simulink model "AM_DSB_TC_PLL"  (R2014b)
settings: Solver=VariableStepDiscrete  StartTime=0.0  StopTime=10  RelTol=1e-3
PreLoadFcn:
  | %%%%%%%%%%%%%%%%%%%%%%%%%%%%%%%%%%%%%%%%%%%%%%%%%%%%%%%%%%%%%%%%%%%%%%%%%%%
  | % check to see if Simulink library folder is missing from the MATLAB path %
  | %%%%%%%%%%%%%%%%%%%%%%%%%%%%%%%%%%%%%%%%%%%%%%%%%%%%%%%%%%%%%%%%%%%%%%%%%%%
  | if isempty(strfind(path, 'rtlsdr_book_library'))
  | 
  |     % create error window
  |     fig_error = figure(...
  |         'Name', 'Error: RTL-SDR Book Library',...
  |         'Toolbar','none',...
  |         'MenuBar','none',...
  |         'NumberTitle','off',...
  |         'Resize','off',...
  |         'WindowStyle','modal');
  |     fig_error.Position(3) = 600;
  |     fig_error.Position(4) = 150;
  |     fig_axes = axes(...
  |         'Parent',fig_error,...
  |         'Position',[0,0,1,1],...
  |         'visible','off');
  |     % error message
  |     t_title = text(.05,.8,...
  |         'MISSING DIRECTORIES',...
  |         'FontSize',11.5);
  |     t_body = text(.075,.6,...
  |         [{'Simulink cannot find the  \it{<root>}\rm / \it{rtlsdr\_book\_library}\rm  folder in the \it{MATLAB Path}\rm.'},...
  |         {'Please set the MATLAB path following the instructions given in Exercise 2.4.'}],...
  |         'FontSize',10.5);
  |     % buttons
  |     btn_path = uicontrol(...
  |         'Parent',fig_error,...
  |         'String','Set Path Now',...
  |         'FontSize',10,...
  |         'Callback', 'pathtool; close(fig_error);',...
  |         'Position', [fig_error.Position(3)/2-210, 30, 200, 30]);
  |     btn_abort = uicontrol(...
  |         'Parent',fig_error,...
  |         'String','No thanks',...
  |         'FontSize',10,...
  |         'Callback', 'close(fig_error); abort=1;',...
  |         'Position', [fig_error.Position(3)/2+10, 30, 200, 30]);
  | 
  |     % pause to allow user to interact with error box
  |     uiwait(fig_error);
  | 
  |     % abort simulation
  |     try
  |         if abort==1
  |             set_param(gcs, 'SimulationCommand', 'stop');
  |         end
  |     end
  | 
  |     % if user has set path, allow diagram to be updated
  |     if ~exist('abort','var')
  |         % create error window
  |         fig_update = figure(...
  |             'Name', 'Update Diagram',...
  |             'Toolbar','none',...
  |             'MenuBar','none',...
  |             'NumberTitle','off',...
  |             'Resize','off');
  |         fig_update.Position(3) = 400;
  |         fig_update.Position(4) = 120;
  |         fig_axes = axes(...
  |             'Parent',fig_update,...
  |             'Position',[0,0,1,1],...
  |             'visible','off');
  |         % instruction message
  |         t_body = text(.075,.7,...
  |             'Once you have set the path, update the block diagram',...
  |             'FontSize',10.5);
  |         % button
  |         btn_update = uicontrol(...
  |             'Parent',fig_update,...
  |             'String','Update Block Diagram',...
  |             'FontSize',10,...
  |             'Callback', 'set_param(gcs,''SimulationCommand'',''update''); close(gcf)',...
  |             'Position', [fig_update.Position(3)/2-100, 30, 200, 30]);
  |     end
  | 
  |     % clear error components
  |     clear('fig_error','fig_update','fig_axes','t_title','t_body','btn_path','btn_abort','btn_update','abort');
  | 
  | end
  | %%%%%%%%%%%%%%%%%%%%%%%%%%%%%%%%%%%%%%%%%%%%%%%%%%%%%%%%%%%%%%%%%%%%%%%%%%%
  | 
  | 
  | fs = 48e3*10;
  | kHz = fs/1000;
  | 
  | fc = fs/5;
  | 
  | % ------- section for synch loop design --------
  | 
  | A = 1;          % assume amplitude of input to PD is 1
  | 
  | T = 1/fs;       % sample period
  | Kp = A/2;      % phase detector is a multiplier
  | Bn = 1000;     % noise bandwidth in Hz
  | Ko = 1;         % gain of NCO (normalised to fs)
  | 
  | d = 0.707;  % damping ratio
  | 
  | % calculate the loop filter coefficients
  | K1 = (4*d*Bn*T)/(Ko*Kp*(d+1/(4*d)));
  | K2 = (4*(Bn*T)^2)/(Ko*Kp*(d+1/4*d)^2);
StopFcn:
  | figure(1)
  | hold off;
  | plot(tx_freq.time,tx_freq.signals.values,'r');
  | hold on;
  | grid on;
  | plot(lo_freq.time,lo_freq.signals.values,'b');
  | xlabel('Time (seconds)');
  | ylabel('Synthesised Frequency (Hz)');
  | legend('Transmitted Carrier','Locally Generated Carrier','location','NorthEast');
  | set(1,'Name','Frequencies of Transmitted and Locally Generated Carriers','NumberTitle','off');
  | setStandardFigSize(1);
undefined symbols (not defined in the file): startfcn_time_scope
libraries: dspmlti4 x6, dspvision x2, commsynccomp2 x2, dsparch4 x1, rtlsdr_book_library x1
CloseFcn:
  | closefcn_model;
Description:
  | Software, Simulation Examples and Design Exercises Licence Agreement
  | 
  | This license agreement refers to the simulation examples, design exercises and files,
  | and associated software MATLAB and Simulink resources that accompany the book:
  | 
  |      Title: Software Defined Radio using MATLAB & Simulink and the RTL-SDR
  |      Published by Strathclyde Academic Media, 2015
  |      Authored by Robert W. Stewart, Kenneth W. Barlee, Dale S.W. Atkinson,
  |      and Louise H. Crockett
  | 
  | and made available as a download from, www.desktopSDR.com or variously acquired
  | by other means such as via USB storage, cloud storage, disk or any other electronic
  | or optical or magnetic storage mechanism. These files and associated software may
  | be used subject to the terms of agreement of the conditions below:
  | 
  |     Copyright © 2015 Robert W. Stewart, Kenneth W. Barlee, Dale S.W. Atkinson,
  |     and Louise H. Crockett
  |     All rights reserved.
  | 
  | Redistribution and use in source and binary forms, with or without modification, are
  | permitted provided that the following conditions are met:
  | 
  |    1.  Redistributions of source code must retain the above copyright notice, this list of
  |         conditions and the following disclaimer.
  | 
  |    2.  Redistributions in binary form must reproduce the above copyright notice, this
  |         list of conditions and the following disclaimer in the documentation and/or other
  |         materials provided with the distribution.
  | 
  |    3.  Neither the name of the copyright holder nor the names of its contributors may
  |         be used to endorse or promote products derived from this software without
  |         specific prior written permission.
  | 
  |    4.  In all cases, the software is, and all modifications and derivatives of the
  |         software shall be, licensed to you solely for use in conjunction with The
  |         MathWorks, Inc. products and service offerings.
  | 
  | THIS SOFTWARE IS PROVIDED BY THE COPYRIGHT HOLDERS AND CONTRIBUTORS
  | "AS IS" AND ANY EXPRESS OR IMPLIED WARRANTIES, INCLUDING, BUT NOT LIMITED
  | TO, THE IMPLIED WARRANTIES OF MERCHANTABILITY AND FITNESS FOR A
  | PARTICULAR PURPOSE ARE DISCLAIMED. IN NO EVENT SHALL THE COPYRIGHT
  | HOLDER OR CONTRIBUTORS BE LIABLE FOR ANY DIRECT, INDIRECT, INCIDENTAL,
  | SPECIAL, EXEMPLARY, OR CONSEQUENTIAL DAMAGES (INCLUDING, BUT NOT
  | LIMITED TO, PROCUREMENT OF SUBSTITUTE GOODS OR SERVICES; LOSS OF USE,
  | DATA, OR PROFITS; OR BUSINESS INTERRUPTION) HOWEVER CAUSED AND ON ANY
  | THEORY OF LIABILITY, WHETHER IN CONTRACT, STRICT LIABILITY, OR TORT
  | (INCLUDING NEGLIGENCE OR OTHERWISE) ARISING IN ANY WAY OUT OF THE USE
  | OF THIS SOFTWARE, EVEN IF ADVISED OF THE POSSIBILITY OF SUCH DAMAGE.
  | 
  | 
  | Audio Tracks used in Simulations Examples and Design Exercises
  | 
  | The music and vocal files used within the Examples files and software within the book
  | were variously written, arranged, performed, recorded and produced by Garrey Rice,
  | Adam Struth, Jamie Struth, Iain Thistlethwaite and also Marshall Craigmyle who
  | collectively, and individually where appropriate, assert and retain all of their copyright,
  | performance and artistic rights. Permission to use and reproduce this music is
  | granted for all purposes associated with MATLAB and Simulink software and the
  | simulation examples and design exercises files that accompany this book. Requests to
  | use the music for any other purpose should be directed to: info@desktopSDR.com.
  | For information on music track names, full credits, and links to the musicians please
  | refer to www.desktopSDR.com/more/audio.
settings Model: Creator=desktopSDR Team  LastModifiedBy=desktopSDR Team
settings DataIOCC: LimitDataPoints=off  SaveOutput=off  SignalLogging=off  SaveTime=off
settings OptimizationCC: InlineParams=on
settings DebuggingCC: ReadBeforeWriteMsg=DisableAll  WriteAfterWriteMsg=DisableAll  WriteAfterReadMsg=DisableAll  UnderspecifiedInitializationDetection=Classic  MergeDetectMultiDrivingBlocksExec=none  MultiTaskDSMMsg=none  ParameterPrecisionLossMsg=none
settings ModelReferenceCC: UpdateModelReferenceTargets=IfOutOfDate
settings SFSimCC: SFSimEcho=off

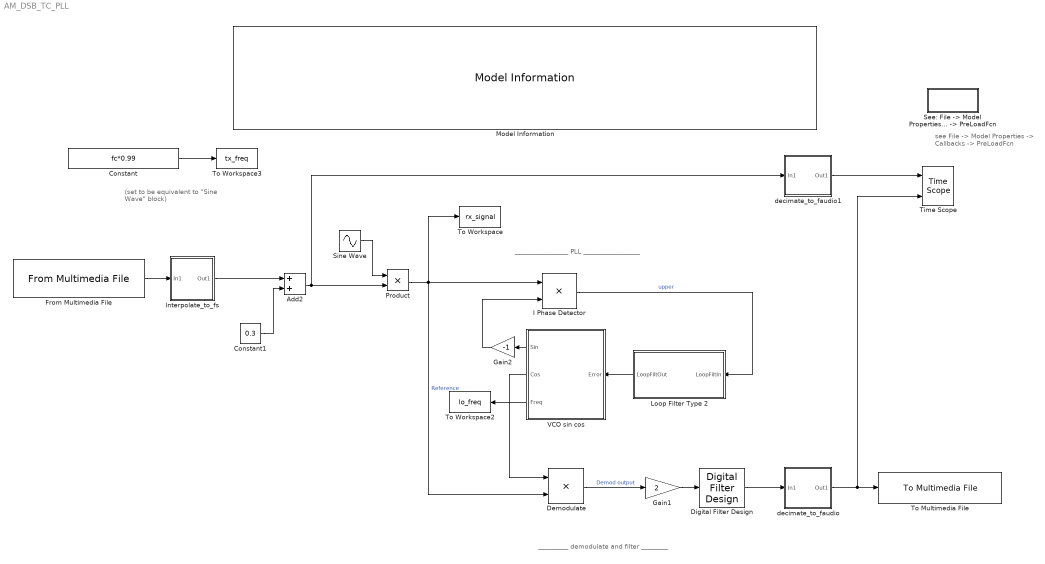
== system AM_DSB_TC_PLL ==
  note: (set to be equivalent to
      | "Sine Wave" block)
  note: ________________ PLL _________________
  note: see File -> Model Properties
      | -> Callbacks -> PreLoadFcn
  note: _________ demodulate and filter ________
  Add2 : Sum
  Constant : Constant  Value=fc*0.99  SampleTime=1/fs
  Constant1 : Constant  Value=0.3  SampleTime=1/fs
  Demodulate : Product
  Digital Filter Design : dsparch4/Digital Filter Design  mwdsp_browser_bugfix_var=off
  From Multimedia File : dspvision/From Multimedia File  inputFilename=..\..\audio_sources\music1_mono48kHz.wav  loop=on  numPlays=inf  outputStreams=Audio only  videoDataType=single  audioDataType=double  inheritSampleTime=on  userDefinedSampleTime=1/30  noAudioOutput=off  isIntensityVideo=off  fourcc=RGB  colorVideoFormat=Separate color signals  outputEOF=off  dataOrg=Column-major  audioFrameSize=600  computeAudioFrameSize=off  outSamplingMode=Frame based
  Gain1 : Gain  Gain=2
  Gain2 : Gain  Gain=-1
  I Phase Detector : Product
  Interpolate_to_fs : Subsystem
  Loop Filter Type 2 : Subsystem  mask(Loop Filter (Type 2)){K1=K1, K2=K2}
      mask prompts: K1 "K1 (proportional path)"; K2 "K2 (integral path)"
      mask help: This loop filter contains two paths: a proportional path with scaling coefficient K1, and an integral path with scaling coefficient K2.
  Model Information : rtlsdr_book_library/Additional Tools/Model Information/Model Information
  Product : Product
  "See: File -> Model Properties -> Callbacks -> PreLoadFcn " : Subsystem
      mask Display:
      | kHz = evalin('base', 'kHz');
      | fprintf(['fs = ',num2str(kHz),' kHz']);
  Sine Wave : Sin  Frequency=2*pi*fc*0.99  Phase=pi/5  SampleTime=1/fs
  Time Scope : TimeScope  StartFcn=startfcn_time_scope;  DefaultConfigurationName=spbscopes.TimeScopeBlockCfg  NumInputPorts=2
  To Multimedia File : dspvision/To Multimedia File  outputFilename=demod_audio_pll.wav  streamSelection=Audio only  videoCompressor=None (uncompressed)  audioCompressor=None (uncompressed)  imagePorts=Separate color signals  fileType=WAV  audioDatatype=16-bit integer  fourcc=RGB  videoQuality=75  mj2000CompFactor=10
  To Workspace : ToWorkspace  VariableName=rx_signal  SaveFormat=Structure With Time  SampleTime=-1
  To Workspace2 : ToWorkspace  VariableName=lo_freq  SaveFormat=Structure With Time  SampleTime=-1
  To Workspace3 : ToWorkspace  VariableName=tx_freq  SaveFormat=Structure With Time  SampleTime=-1
  VCO sin cos : Subsystem  mask(Quadratude VCO){fq=fc, sensitivity=Ko*fs}
      mask prompts: fq "Quiescent Frequency (Hz)"; sensitivity "Sensitivity (Hz/V)"
      mask help: This VCO provides both cosine and sine outputs. The quiescent frequency and sensitivity of the VCO can be defined via the mask (and these apply to both sine and cosine outputs). The block also provides the instantaneous frequency as an output.
  decimate_to_faudio : Subsystem
  decimate_to_faudio1 : Subsystem
  wires:
  Sine Wave/1 -> Product/1
  Product/1 -> Demodulate/2, To Workspace/1, I Phase Detector/1  "Reference"
  Demodulate/1 -> Gain1/1  "Demod output"
  From Multimedia File/1 -> Interpolate_to_fs/1(In1)
  I Phase Detector/1 -> Loop Filter Type 2/1(LoopFiltIn)  "upper"
  Gain2/1 -> I Phase Detector/2
  VCO sin cos/3(Freq) -> To Workspace2/1
  Constant/1 -> To Workspace3/1
  Constant1/1 -> Add2/2
  Interpolate_to_fs/1(Out1) -> Add2/1
  decimate_to_faudio/1(Out1) -> Time Scope/2, To Multimedia File/1
  Digital Filter Design/1 -> decimate_to_faudio/1(In1)
  VCO sin cos/2(Cos) -> Demodulate/1
  Add2/1 -> decimate_to_faudio1/1(In1), Product/2
  decimate_to_faudio1/1(Out1) -> Time Scope/1
  Gain1/1 -> Digital Filter Design/1
  VCO sin cos/1(Sin) -> Gain2/1
  Loop Filter Type 2/1(LoopFiltOut) -> VCO sin cos/1(Error)

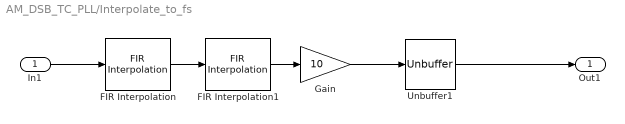
== system AM_DSB_TC_PLL/Interpolate_to_fs ==
  In1 : Inport
  FIR Interpolation : dspmlti4/FIR Interpolation  h=fir1(35,1/5)  L=5  framing=Allow multirate processing  outputBufInitCond=0  InputProcessing=Columns as channels (frame based)  firstCoeffDataTypeStr=Inherit: Same word length as input  firstCoeffLastDataTypeStr=Inherit: Same word length as input  firstCoeffMin=[]  firstCoeffMax=[]  outputDataTypeStr=Inherit: Same as accumulator  outputLastDataTypeStr=Inherit: Same as accumulator  outputMin=[]  outputMax=[]  roundingMode=Floor  overflowMode=off  FilterSource=Specify via dialog  FilterObject=Hm_firinterp
  FIR Interpolation1 : dspmlti4/FIR Interpolation  h=fir1(35,1/2)  L=2  framing=Allow multirate processing  outputBufInitCond=0  InputProcessing=Columns as channels (frame based)  firstCoeffDataTypeStr=Inherit: Same word length as input  firstCoeffLastDataTypeStr=Inherit: Same word length as input  firstCoeffMin=[]  firstCoeffMax=[]  outputDataTypeStr=Inherit: Same as accumulator  outputLastDataTypeStr=Inherit: Same as accumulator  outputMin=[]  outputMax=[]  roundingMode=Floor  overflowMode=off  FilterSource=Specify via dialog  FilterObject=Hm_firinterp
  Gain : Gain  Gain=10
  Unbuffer1 : Unbuffer  SampleBasedProcessing=Same as frame based
  Out1 : Outport
  wires:
  FIR Interpolation/1 -> FIR Interpolation1/1
  FIR Interpolation1/1 -> Gain/1
  In1/1 -> FIR Interpolation/1
  Gain/1 -> Unbuffer1/1
  Unbuffer1/1 -> Out1/1

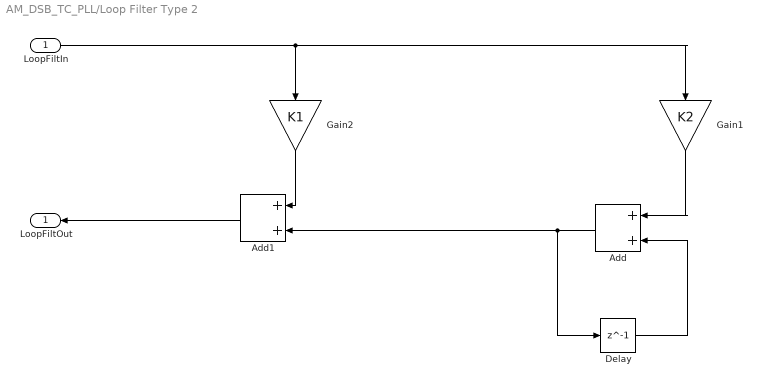
== system AM_DSB_TC_PLL/Loop Filter Type 2 ==
  LoopFiltIn : Inport
  Add : Sum
  Add1 : Sum
  Delay : Delay  DelayLength=1
  Gain1 : Gain  Gain=K2
  Gain2 : Gain  Gain=K1
  LoopFiltOut : Outport
  wires:
  Add1/1 -> LoopFiltOut/1
  Delay/1 -> Add/2
  Add/1 -> Delay/1, Add1/2
  LoopFiltIn/1 -> Gain2/1, Gain1/1
  Gain2/1 -> Add1/1
  Gain1/1 -> Add/1

== system AM_DSB_TC_PLL/See: File -> Model Properties -> Callbacks -> PreLoadFcn  ==

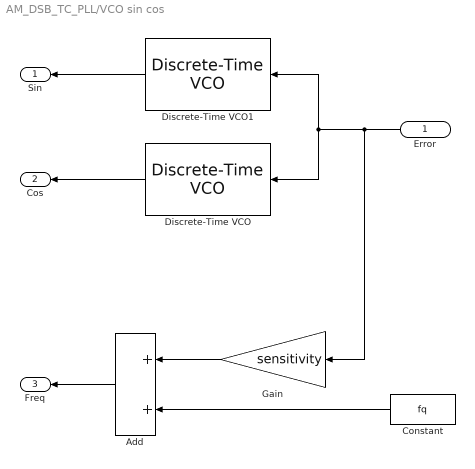
== system AM_DSB_TC_PLL/VCO sin cos ==
  Error : Inport
  Add : Sum
  Constant : Constant  Value=fq  SampleTime=1/fs
  Discrete-Time VCO : commsynccomp2/Discrete-Time VCO  Ac=1  Fc=fq  Kc=sensitivity  Ph=pi/2  ts=1/fs
  Discrete-Time VCO1 : commsynccomp2/Discrete-Time VCO  Ac=1  Fc=fq  Kc=sensitivity  Ph=0  ts=1/fs
  Gain : Gain  Gain=sensitivity
  Sin : Outport
  Cos : Outport  Port=2
  Freq : Outport  Port=3
  wires:
  Discrete-Time VCO1/1 -> Sin/1
  Discrete-Time VCO/1 -> Cos/1
  Error/1 -> Gain/1, Discrete-Time VCO/1, Discrete-Time VCO1/1
  Gain/1 -> Add/1
  Constant/1 -> Add/2
  Add/1 -> Freq/1

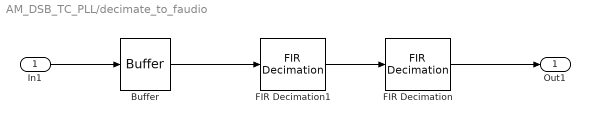
== system AM_DSB_TC_PLL/decimate_to_faudio ==
  In1 : Inport
  Buffer : Buffer  TreatMby1Signals=One channel
  FIR Decimation : dspmlti4/FIR Decimation  h=fir1(35,1/5)  D=5  filtStruct=Direct form  framing=Allow multirate processing  inputOffset=0  outputBufInitCond=0  InputProcessing=Columns as channels (frame based)  firstCoeffDataTypeStr=Inherit: Same word length as input  firstCoeffLastDataTypeStr=Inherit: Same word length as input  firstCoeffMin=[]  firstCoeffMax=[]  outputDataTypeStr=Inherit: Same as accumulator  outputLastDataTypeStr=Inherit: Same as accumulator  outputMin=[]  outputMax=[]  roundingMode=Floor  overflowMode=off  FilterSource=Specify via dialog  FilterObject=Hm_firdecim
      settings: allowOverrides=off
  FIR Decimation1 : dspmlti4/FIR Decimation  h=fir1(35,1/2)  D=2  filtStruct=Direct form  framing=Allow multirate processing  inputOffset=0  outputBufInitCond=0  InputProcessing=Columns as channels (frame based)  firstCoeffDataTypeStr=Inherit: Same word length as input  firstCoeffLastDataTypeStr=Inherit: Same word length as input  firstCoeffMin=[]  firstCoeffMax=[]  outputDataTypeStr=Inherit: Same as accumulator  outputLastDataTypeStr=Inherit: Same as accumulator  outputMin=[]  outputMax=[]  roundingMode=Floor  overflowMode=off  FilterSource=Specify via dialog  FilterObject=Hm_firdecim
      settings: allowOverrides=off
  Out1 : Outport
  wires:
  FIR Decimation/1 -> Out1/1
  FIR Decimation1/1 -> FIR Decimation/1
  Buffer/1 -> FIR Decimation1/1
  In1/1 -> Buffer/1

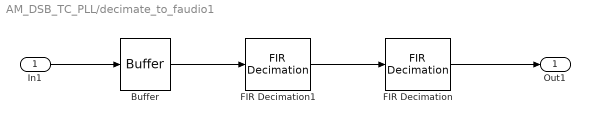
== system AM_DSB_TC_PLL/decimate_to_faudio1 ==
  In1 : Inport
  Buffer : Buffer  TreatMby1Signals=One channel
  FIR Decimation : dspmlti4/FIR Decimation  h=fir1(35,1/5)  D=5  filtStruct=Direct form  framing=Allow multirate processing  inputOffset=0  outputBufInitCond=0  InputProcessing=Columns as channels (frame based)  firstCoeffDataTypeStr=Inherit: Same word length as input  firstCoeffLastDataTypeStr=Inherit: Same word length as input  firstCoeffMin=[]  firstCoeffMax=[]  outputDataTypeStr=Inherit: Same as accumulator  outputLastDataTypeStr=Inherit: Same as accumulator  outputMin=[]  outputMax=[]  roundingMode=Floor  overflowMode=off  FilterSource=Specify via dialog  FilterObject=Hm_firdecim
      settings: allowOverrides=off
  FIR Decimation1 : dspmlti4/FIR Decimation  h=fir1(35,1/2)  D=2  filtStruct=Direct form  framing=Allow multirate processing  inputOffset=0  outputBufInitCond=0  InputProcessing=Columns as channels (frame based)  firstCoeffDataTypeStr=Inherit: Same word length as input  firstCoeffLastDataTypeStr=Inherit: Same word length as input  firstCoeffMin=[]  firstCoeffMax=[]  outputDataTypeStr=Inherit: Same as accumulator  outputLastDataTypeStr=Inherit: Same as accumulator  outputMin=[]  outputMax=[]  roundingMode=Floor  overflowMode=off  FilterSource=Specify via dialog  FilterObject=Hm_firdecim
      settings: allowOverrides=off
  Out1 : Outport
  wires:
  In1/1 -> Buffer/1
  Buffer/1 -> FIR Decimation1/1
  FIR Decimation1/1 -> FIR Decimation/1
  FIR Decimation/1 -> Out1/1
